simulink model "demoqp"  (R2020b)
settings: Solver=VariableStepAuto  StartTime=0.0  StopTime=10.0  RelTol=1e-3
settings Model: Creator=abhis  LastModifiedBy=abhis

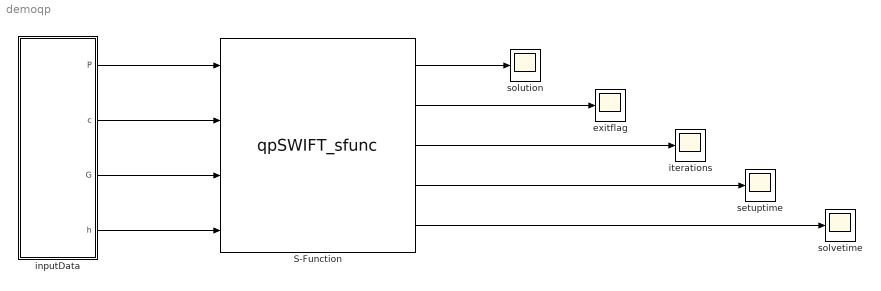
== system demoqp ==
  S-Function : S-Function  FunctionName=qpSWIFT_sfunc  SFunctionDeploymentMode=off  EnableBusSupport=off
  exitflag : Scope
  inputData : MATLAB Function  TreatAsAtomicUnit=on
  iterations : Scope
  setuptime : Scope
  solution : Scope
  solvetime : Scope
  wires:
  inputData/1(P) -> S-Function/1
  inputData/2(c) -> S-Function/2
  inputData/3(G) -> S-Function/3
  inputData/4(h) -> S-Function/4
  S-Function/4 -> setuptime/1
  S-Function/1 -> solution/1
  S-Function/5 -> solvetime/1
  S-Function/2 -> exitflag/1
  S-Function/3 -> iterations/1

== matlab function demoqp/inputData ==
  data: P output; c output; G output; h output
function [P,c,G,h] = fcn()


%%%% Cost Function
in_P = [5 1 0; 1 2 1; 0 1 4];
c = [1; 2; 1];



%%%% Inequality Constraints
in_G = [-4 -4 0; 0 0 -1];
h = [-1; -1];


P = in_P(:);
G = in_G(:);


end
